simulink model "Ventilator_Controller"  (R2019b)
settings: Solver=ode23tb  StartTime=0  StopTime=1000  FixedStep=0.001  MaxStep=time_step_new  RelTol=0.01  EnableMultiTasking=on
values from neighbouring files (symbols this model uses):
  A = 20.9    [Gas_Exchange_IC.m]    (also in getPneumonia.m = (LF1-LF2)/(1-exp(Rresolve*(t2(end)-t2(1)))))
  a1 = 0.3836    [Dissociation_Spencer_IC.m]    (also in Gas_Exchange_IC.m; Respiratory_IC.m)
  a2 = 1.819    [Dissociation_Spencer_IC.m]    (also in Gas_Exchange_IC.m; Respiratory_IC.m)
  alpha1 = 0.02598    [Dissociation_Spencer_IC.m]    (also in Gas_Exchange_IC.m; Respiratory_IC.m)
  alpha2 = 0.05591    [Dissociation_Spencer_IC.m]    (also in Gas_Exchange_IC.m; Respiratory_IC.m)
  B = 92.8    [Gas_Exchange_IC.m]    (also in getPneumonia.m = LungFunction(end)-A)
  beta1 = 0.012275    [Dissociation_Spencer_IC.m]    (also in Gas_Exchange_IC.m; Respiratory_IC.m)
  beta2 = 0.03255    [Dissociation_Spencer_IC.m]    (also in Gas_Exchange_IC.m; Respiratory_IC.m)
  C = 10570    [Gas_Exchange_IC.m]
  C1 = 9    [Dissociation_Spencer_IC.m]    (also in Gas_Exchange_IC.m; Respiratory_IC.m)
  C2 = 87.00    (= 87)    [Dissociation_Spencer_IC.m]    (also in Gas_Exchange_IC.m; Respiratory_IC.m)
  Circadian_Period = 24    [Respiratory_IC.m]    (also in State_UA_Khoo_IC.m)
  CvCO2IC = 0.5116    [Body_Khoo_IC.m]    (also in Gas_Exchange_IC.m; Respiratory_IC.m = 0.5247)
  CvO2IC = 0.1672    [Body_Khoo_IC.m]    (also in Gas_Exchange_IC.m; Respiratory_IC.m = 0.1639)
  D = -5.251    [Gas_Exchange_IC.m]
  Dead1CO2IC = 0.1020    (= 0.102)    [Dead_Space_Khoo_IC.m]    (also in Gas_Exchange_IC.m; Respiratory_IC.m = 39.5616)
  Dead1O2IC = 149.8824    [Dead_Space_Khoo_IC.m]    (also in Gas_Exchange_IC.m; Respiratory_IC.m = 104.3637)
  Dead2CO2IC = 0.5274    [Dead_Space_Khoo_IC.m]    (also in Gas_Exchange_IC.m; Respiratory_IC.m = 39.6736)
  Dead2O2IC = 149.3923    [Dead_Space_Khoo_IC.m]    (also in Gas_Exchange_IC.m; Respiratory_IC.m = 104.2258)
  Dead3CO2IC = 2.2996    [Dead_Space_Khoo_IC.m]    (also in Gas_Exchange_IC.m; Respiratory_IC.m = 39.8127)
  Dead3O2IC = 147.3503    [Dead_Space_Khoo_IC.m]    (also in Gas_Exchange_IC.m; Respiratory_IC.m = 104.0505)
  Dead4CO2IC = 8.2293    [Dead_Space_Khoo_IC.m]    (also in Gas_Exchange_IC.m; Respiratory_IC.m = 40.0061)
  Dead4O2IC = 140.5179    [Dead_Space_Khoo_IC.m]    (also in Gas_Exchange_IC.m; Respiratory_IC.m = 103.8005)
  Dead5CO2IC = 22.0757    [Dead_Space_Khoo_IC.m]    (also in Gas_Exchange_IC.m; Respiratory_IC.m = 40.3359)
  Dead5O2IC = 124.5641    [Dead_Space_Khoo_IC.m]    (also in Gas_Exchange_IC.m; Respiratory_IC.m = 103.3579)
  DtotalIC = 0.3    [NeuroMuscular_IC.m]    (also in Respiratory_IC.m = 0.32)
  E_CW = 5    [Pleural_Schuessler_IC.m]    (also in Pmus_Flow_Younes_IC.m; Resp_Mech_IC.m; Respiratory_IC.m)
  E_L = 5    [Pleural_Schuessler_IC.m]    (also in Pmus_Flow_Younes_IC.m; Resp_Mech_IC.m; Respiratory_IC.m)
  fc = 0.4/60    (= 0.00666666666667)    [Respiratory_IC.m]    (also in State_UA_Khoo_IC.m)
  fcs_max = 47.78    [Cardiovascular_IC.m]    (also in Reflex_Ursino_IC.m)
  fcs_min = 2.52    [Cardiovascular_IC.m]    (also in Reflex_Ursino_IC.m)
  fcs_zero = 25    [Respiratory_IC.m]
  FlowIC = 0    [Pmus_Flow_Younes_IC.m]    (also in Resp_Mech_IC.m; Respiratory_IC.m)
  fp_inf = 6.3    [Respiratory_IC.m]
  fp_zero = 3.2    [Respiratory_IC.m]
  fs_inf = 2.10    (= 2.1)    [Respiratory_IC.m]
  fs_zero = 16.11    [Respiratory_IC.m]
  ftbs_min = 0.1    [Cardiovascular_IC.m]    (also in SA_Node_Ursino_IC.m)
  gc = 0.008/60    (= 0.000133333333333)    [Respiratory_IC.m]    (also in State_UA_Khoo_IC.m)
  h = 0.0183    [Brain_Khoo_IC.m]    (also in Gas_Exchange_IC.m; Respiratory_IC.m)
  HP_basal = 0.58    [Cardiovascular_IC.m]    (also in SA_Node_Ursino_IC.m)
  Ic = 45    [Gas_Exchange_IC.m]    (also in Respiratory_IC.m; Vent_Drive_Khoo_IC.m)
  IpCO2 = 38    [Gas_Exchange_IC.m]    (also in Respiratory_IC.m; Vent_Drive_Khoo_IC.m)
  IpO2 = 102.4    [Gas_Exchange_IC.m]    (also in Respiratory_IC.m; Vent_Drive_Khoo_IC.m)
  K1 = 13    [Dissociation_Spencer_IC.m]    (also in Gas_Exchange_IC.m; Respiratory_IC.m)
  K2 = 194.4    [Dissociation_Spencer_IC.m]    (also in Gas_Exchange_IC.m; Respiratory_IC.m)
  k_cs = 11.758    [Cardiovascular_IC.m]    (also in Reflex_Ursino_IC.m)
  k_p = 7.06    [Respiratory_IC.m]
  k_s = 0.07    [Respiratory_IC.m]
  lambda = 863    [Gas_Exchange_IC.m]    (also in Lungs_Khoo_IC.m; Respiratory_IC.m)
  Mech_Vent_pressure = 17    [Mech_vent_test.m]
  MRbCO2 = 0.0517    [Brain_Khoo_IC.m]    (also in Gas_Exchange_IC.m; Respiratory_IC.m)
  MRCO2 = 0.0033    [Body_Khoo_IC.m]    (also in Gas_Exchange_IC.m; Respiratory_IC.m)
  MRO2 = 0.0038    [Body_Khoo_IC.m]    (also in Gas_Exchange_IC.m; Respiratory_IC.m)
  NM_block_gain = 1    [Mech_vent_test.m]
  PACO2_delayIC = 39.6041    [Cardio_Mix_Lange_IC.m]    (also in Gas_Exchange_IC.m; Respiratory_IC.m = 40.4448)
  PaCO2firstIC = 0.2150    (= 0.215)    [Cardio_Mix_Lange_IC.m]    (also in Gas_Exchange_IC.m; Respiratory_IC.m = -0.2465)
  PACO2IC = 37.1484    [Gas_Exchange_IC.m]    (also in Lungs_Khoo_IC.m; Respiratory_IC.m = 40.9432)
  PaCO2secondIC = 38.4577    [Cardio_Mix_Lange_IC.m]    (also in Gas_Exchange_IC.m; Respiratory_IC.m = 40.3928)
  PAO2_delayIC = 103.8436    [Cardio_Mix_Lange_IC.m]    (also in Gas_Exchange_IC.m; Respiratory_IC.m = 103.1223)
  PaO2firstIC = -0.2838    [Cardio_Mix_Lange_IC.m]    (also in Gas_Exchange_IC.m; Respiratory_IC.m = 0.3557)
  PAO2IC = 107.1983    [Gas_Exchange_IC.m]    (also in Lungs_Khoo_IC.m; Respiratory_IC.m = 102.5153)
  PaO2secondIC = 105.4828    [Cardio_Mix_Lange_IC.m]    (also in Gas_Exchange_IC.m; Respiratory_IC.m = 103.1435)
  PbCO2IC = 48.2858    [Brain_Khoo_IC.m]    (also in Gas_Exchange_IC.m; Respiratory_IC.m = 48.5383)
  PICO2 = 0    [Dead_Space_Khoo_IC.m]    (also in Gas_Exchange_IC.m; Respiratory_IC.m)
  PICO2_change = 0    [Respiratory_IC.m]
  PIO2 = 150    [Dead_Space_Khoo_IC.m]    (also in Gas_Exchange_IC.m; Respiratory_IC.m)
  PIO2_change = -90    [Mech_vent_test.m]    (also in Respiratory_IC.m = 0)
  Pn = 90    [Cardiovascular_IC.m]    (also in Reflex_Ursino_IC.m)
  Pt_frcIC1 = 0    [Pmus_Flow_Younes_IC.m]    (also in Resp_Mech_IC.m; Respiratory_IC.m)
  Pt_frcIC2 = 0    [Pmus_Flow_Younes_IC.m]    (also in Resp_Mech_IC.m; Respiratory_IC.m)
  QdBo = 0.8333    [Brain_Khoo_IC.m]    (also in Gas_Exchange_IC.m; Respiratory_IC.m)
  R_AW = 1.27    [Pleural_Schuessler_IC.m]    (also in Pmus_Flow_Younes_IC.m; Resp_Mech_IC.m; Respiratory_IC.m)
  R_CW = 1.03    [Pleural_Schuessler_IC.m]    (also in Pmus_Flow_Younes_IC.m; Resp_Mech_IC.m; Respiratory_IC.m)
  R_L = 1.69    [Pleural_Schuessler_IC.m]    (also in Pmus_Flow_Younes_IC.m; Resp_Mech_IC.m; Respiratory_IC.m)
  RC = 0.06    [Pleural_Schuessler_IC.m]    (also in Pmus_Flow_Younes_IC.m; Resp_Mech_IC.m; Respiratory_IC.m)
  rc = 0.2/60    (= 0.00333333333333)    [Respiratory_IC.m]    (also in State_UA_Khoo_IC.m)
  SbCO2 = 0.3600    (= 0.36)    [Brain_Khoo_IC.m]    (also in Gas_Exchange_IC.m; Respiratory_IC.m)
  SCO2 = 0.0043    [Brain_Khoo_IC.m]    (also in Gas_Exchange_IC.m; Respiratory_IC.m)
  SWAo = 0.007    [Respiratory_IC.m]    (also in State_UA_Khoo_IC.m)
  T1 = 1    [Cardio_Mix_Lange_IC.m]    (also in Gas_Exchange_IC.m; Respiratory_IC.m)
  T2 = 2    [Cardio_Mix_Lange_IC.m]    (also in Gas_Exchange_IC.m; Respiratory_IC.m)
  t_CO2_duration = 0    [Respiratory_IC.m]
  t_CO2_start = 0    [Respiratory_IC.m]
  t_end_new = 4*24*60*60    (= 345600)    [Mech_vent_test.m]
  t_end_UA = 0    [Respiratory_IC.m]    (also in State_UA_Khoo_IC.m)
  t_Mech_Vent_duration = 0    [Mech_vent_test.m]
  t_Mech_Vent_start = 0    [Mech_vent_test.m]
  t_Mueller_duration = 0    [NeuroMuscular_IC.m]
  t_Mueller_insp = 0    [NeuroMuscular_IC.m]
  t_Mueller_start = 0    [NeuroMuscular_IC.m]
  t_NM_block_duration = 0    [Mech_vent_test.m]
  t_NM_block_start = 0    [Mech_vent_test.m]
  t_O2_duration = 0    [Mech_vent_test.m]    (also in Respiratory_IC.m)
  t_O2_start = 0    [Mech_vent_test.m]    (also in Respiratory_IC.m)
  t_start_new = 0    [Mech_vent_test.m]
  t_start_UA = 0    [Respiratory_IC.m]    (also in State_UA_Khoo_IC.m)
  t_valsalva_duration = 0    [NeuroMuscular_IC.m]
  t_valsalva_insp = 0    [NeuroMuscular_IC.m]
  t_valsalva_start = 0    [NeuroMuscular_IC.m]
  time_step = time_step    [acquire_data.m]    (also in acquire_data_save.m)
  VC = 5    [Pmus_Flow_Younes_IC.m]    (also in Resp_Mech_IC.m; Respiratory_IC.m)
  Vdead1 = 0.03    [Dead_Space_Khoo_IC.m]    (also in Gas_Exchange_IC.m; Respiratory_IC.m)
  Vdead2 = 0.03    [Dead_Space_Khoo_IC.m]    (also in Gas_Exchange_IC.m; Respiratory_IC.m)
  Vdead3 = 0.03    [Dead_Space_Khoo_IC.m]    (also in Gas_Exchange_IC.m; Respiratory_IC.m)
  Vdead4 = 0.03    [Dead_Space_Khoo_IC.m]    (also in Gas_Exchange_IC.m; Respiratory_IC.m)
  Vdead5 = 0.03    [Dead_Space_Khoo_IC.m]    (also in Gas_Exchange_IC.m; Respiratory_IC.m)
  Ventilator_rate = 12    [Mech_vent_test.m]
  VTCO2 = 15    [Body_Khoo_IC.m]    (also in Gas_Exchange_IC.m; Respiratory_IC.m)
  VtIC = 0    [Pmus_Flow_Younes_IC.m]    (also in Resp_Mech_IC.m; Respiratory_IC.m)
  VTO2 = 6    [Body_Khoo_IC.m]    (also in Gas_Exchange_IC.m; Respiratory_IC.m)
  Z = 0.0227    [Dissociation_Spencer_IC.m]    (also in Gas_Exchange_IC.m; Respiratory_IC.m)
undefined symbols (not defined in the file or in its folder): A_0_ua, alpha_E_FFA_Heart, alpha_E_FFA_muscle, alpha_E_GLC_Heart, alpha_E_GLC_muscle, alpha_E_GLY_muscle, alpha_E_PYR_muscle, alpha_E_TGL_adipose, alpha_E_TGL_GI, alpha_E_TGL_Heart, alpha_E_TGL_muscle, Arousal_UAIC, C_ua_awake, Cbp, Cbv, Ce_0, Cep, Cev, Chp, Chv, Cla, Clamp_class, Cmp, Cmv, Cpa, CPAP_pressure, Cpp, Cpv, Cra, Csa, Csp, Csv, CvbO2_n, CvhO2_n, CvmO2_n, DAY, delay, DietBlock, Dx, Fb, fchemo_max, fchemo_min, fchemoIC, flsIC, Ftas_I0, ftas_min, ftas_r0, FVC_activation, gain_E, Gamma, Gas_sleep, Gas_sleepM, Gb, Gblock, GbO2, Gbs_sleep, gcc_sa, gcc_sb, gcc_sp, Gclamp ... (+147)
libraries: simulink x4, simulink_extras x2
(part 1 of 8)
settings Model: SimulationMode=accelerator  ExtModeTrigMode=oneshot  ExtModeArmWhenConnect=off  Creator=cPhonix  LastModifiedBy=z9070419
settings SolverCC: MaxConsecutiveZCs=10000  AutoInsertRateTranBlk=on
settings DataIOCC: FinalStateName=yFinal  InitialState=xFinal  SaveFormat=Array  SaveOutput=off  SaveTime=off  ReturnWorkspaceOutputs=off  TimeSaveName=T_SIMULATION  SignalLoggingName=sigsOut
settings OptimizationCC: BlockReduction=off  BooleanDataType=off  ExpressionDepthLimit=2147483647  InitFltsAndDblsToZero=on  LifeSpan=inf
settings DebuggingCC: AlgebraicLoopMsg=error  ArtificialAlgebraicLoopMsg=error  SaveWithParameterizedLinksMsg=none  UnderspecifiedInitializationDetection=Classic  MergeDetectMultiDrivingBlocksExec=none  SignalResolutionControl=TryResolveAllWithWarning  InheritedTsInSrcMsg=none  MultiTaskDSMMsg=warning  MultiTaskCondExecSysMsg=none  MultiTaskRateTransMsg=warning  TasksWithSamePriorityMsg=none  SigSpecEnsureSampleTimeMsg=none  IntegerOverflowMsg=none  Int32ToFloatConvMsg=none  ParameterDowncastMsg=warning  ParameterOverflowMsg=none  FcnCallInpInsideContextMsg=warning  ModelReferenceDataLoggingMessage=none  StateNameClashWarn=warning  SFUnexpectedBacktrackingDiag=warning  SFNoUnconditionalDefaultTransitionDiag=warning  SFExecutionAtInitializationDiag=none  IntegerSaturationMsg=none  ArithmeticOperatorsInVariantConditions=warning
settings HardwareCC: ProdBitPerPointer=32  ProdBitPerSizeT=32  ProdBitPerPtrDiffT=32  ProdLargestAtomicFloat=None  ProdIntDivRoundTo=Undefined  ProdEndianess=Unspecified  ProdWordSize=32  ProdHWDeviceType=32-bit Generic  TargetBitPerPointer=64  TargetBitPerSizeT=64  TargetBitPerPtrDiffT=64  TargetLongLongMode=on  TargetIntDivRoundTo=Zero  TargetEndianess=LittleEndian  TargetWordSize=64  TargetHWDeviceType=MATLAB Host  ProdEqTarget=off
settings ModelReferenceCC: PropagateSignalLabelsOutOfModel=off
settings SFSimCC: SimParseCustomCode=off
settings CodeAppCC: StateflowObjectComments=on
settings GRTTargetCC: TargetLangStandard=C89/C90 (ANSI)  CombineOutputUpdateFcns=off  GRTInterface=on
settings ConfigComp: CovMetricSettings=dw  CovHtmlReporting=on  CovSaveCumulativeToWorkspaceVar=on  CovSaveSingleToWorkspaceVar=on

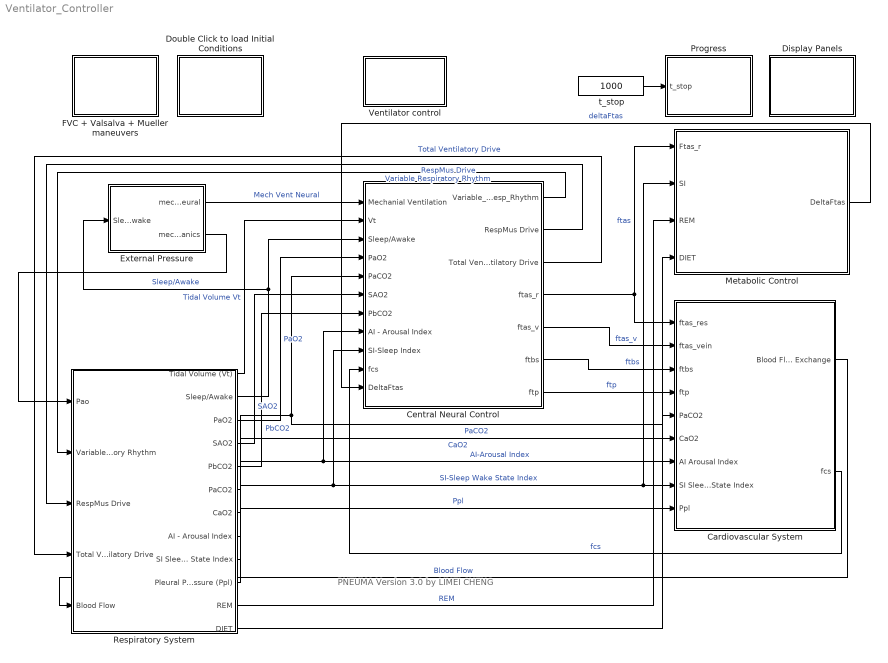
== system Ventilator_Controller ==
  note: PNEUMA Version 3.0 by LIMEI CHENG
  Cardiovascular System : Subsystem
      mask Display: image(imread('CV_pic.bmp'))
  Central Neural Control : Subsystem
      mask Display: image(imread('CNS.bmp'))
  Display Panels : Subsystem
      mask Display: disp('Display \nPanel','b')
  Double Click to load Initial Conditions : Subsystem
      settings: OpenFcn=pneuma_variables
      mask Display: image(imread('IC_pic.bmp'))
  External Pressure : Subsystem
      mask Display: image(imread('CPAP2.bmp'))
  FVC + Valsalva + Mueller maneuvers : Subsystem
      mask Display: disp('Maneuvers')
  Metabolic Control : Subsystem
      mask Display: image(imread('Metabolic2.bmp'))
  Progress : Subsystem
      mask Display: disp('Progress')
  Respiratory System : Subsystem
      mask Display: image(imread('Respiratory_System.bmp'))
  Ventilator control : Subsystem
  t_stop : Constant  Value=1000
  wires:
  Central Neural Control/3(Total Ventilatory Drive) -> Respiratory System/4(Total Ventilatory Drive)  "Total Ventilatory Drive"
  Central Neural Control/2(RespMus Drive) -> Respiratory System/3(RespMus Drive)  "RespMus Drive"
  External Pressure/1(mech vent neural) -> Central Neural Control/1(Mechanial Ventilation)  "Mech Vent Neural"
  Cardiovascular System/1(Blood Flow to Lung for Gas Exchange) -> Respiratory System/5(Blood Flow)  "Blood Flow"
  Cardiovascular System/2(fcs) -> Central Neural Control/10(fcs)  "fcs"
  t_stop/1 -> Progress/1(t_stop)
  Central Neural Control/1(Variable_Resp_Rhythm) -> Respiratory System/2(Variable Respiratory Rhythm)  "Variable Respiratory Rhythm"
  Respiratory System/1(Tidal Volume (Vt)) -> Central Neural Control/2(Vt)  "Tidal Volume Vt"
  Respiratory System/2(Sleep/Awake) -> Central Neural Control/3(Sleep/Awake), External Pressure/1(SleepAwake)  "Sleep/Awake"
  Respiratory System/3(PaO2) -> Central Neural Control/4(PaO2)  "PaO2"
  Respiratory System/6(PaCO2) -> Central Neural Control/5(PaCO2), Cardiovascular System/5(PaCO2)  "PaCO2"
  Respiratory System/4(SAO2) -> Central Neural Control/6(SAO2)  "SAO2"
  Respiratory System/5(PbCO2) -> Central Neural Control/7(PbCO2)  "PbCO2"
  Respiratory System/8(AI - Arousal Index) -> Central Neural Control/8(AI - Arousal Index), Cardiovascular System/7(AI Arousal Index)  "AI-Arousal Index"
  Respiratory System/9(SI Sleep Wake State Index) -> Metabolic Control/2(SI), Cardiovascular System/8(SI Sleep-Wake State Index), Central Neural Control/9(SI-Sleep Index)  "SI-Sleep Wake State Index"
  Respiratory System/10(Pleural Pressure (Ppl)) -> Cardiovascular System/9(Ppl)  "Ppl"
  External Pressure/2(mech vent mechanics) -> Respiratory System/1(Pao)
  Respiratory System/7(CaO2) -> Cardiovascular System/6(CaO2)  "CaO2"
  Central Neural Control/4(ftas_r) -> Metabolic Control/1(Ftas_r), Cardiovascular System/1(ftas_res)  "ftas"
  Central Neural Control/5(ftas_v) -> Cardiovascular System/2(ftas_vein)  "ftas_v"
  Central Neural Control/6(ftbs) -> Cardiovascular System/3(ftbs)  "ftbs"
  Central Neural Control/7(ftp) -> Cardiovascular System/4(ftp)  "ftp"
  Respiratory System/11(REM) -> Metabolic Control/3(REM)  "REM"
  Metabolic Control/1(DeltaFtas) -> Central Neural Control/11(DeltaFtas)  "deltaFtas"
  Respiratory System/12(DIET) -> Metabolic Control/4(DIET)

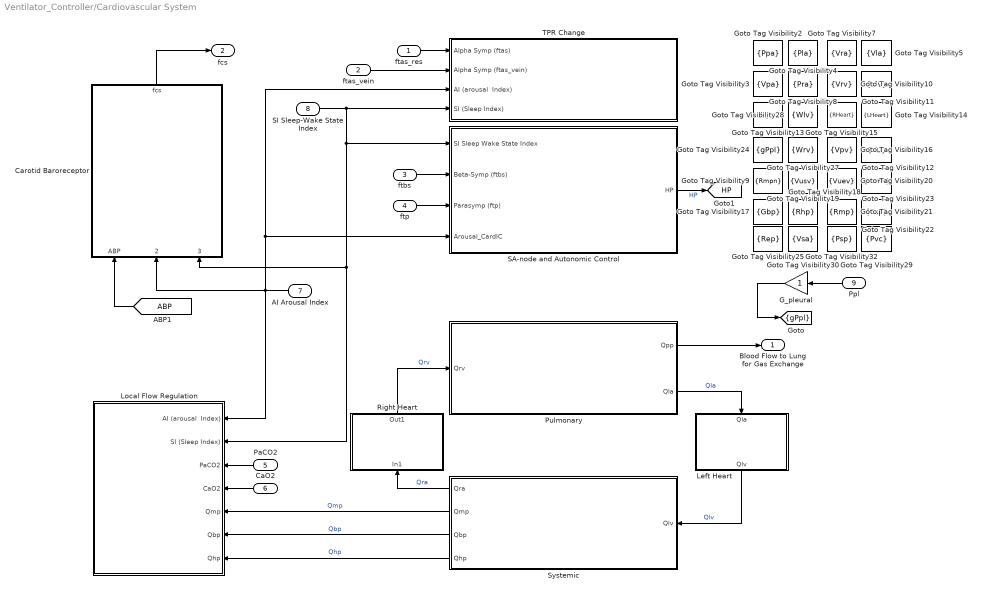
== system Ventilator_Controller/Cardiovascular System ==
  ftas_res : Inport
  ftas_vein : Inport  Port=2
  ftbs : Inport  Port=3
  ftp : Inport  Port=4
  PaCO2 : Inport  Port=5
  CaO2 : Inport  Port=6
  AI Arousal Index : Inport  Port=7  OutDataTypeStr=double
  SI Sleep-Wake State Index : Inport  Port=8
  Ppl : Inport  Port=9
  Carotid Baroreceptor : Subsystem
      mask Display: disp('Carotid\n Baroreceptor')
  G_pleural : Gain  SaturateOnIntegerOverflow=on  OutDataTypeStr=Inherit: Same as input  ParamDataTypeStr=Inherit: Same as input
  Goto Tag Visibility10 : GotoTagVisibility  GotoTag=Vrv
  Goto Tag Visibility11 : GotoTagVisibility  GotoTag=Vlv
  Goto Tag Visibility12 : GotoTagVisibility  GotoTag=Vu
  Goto Tag Visibility13 : GotoTagVisibility  GotoTag=Vpp
  Goto Tag Visibility14 : GotoTagVisibility  GotoTag=LHeart
  Goto Tag Visibility15 : GotoTagVisibility  GotoTag=RHeart
  Goto Tag Visibility16 : GotoTagVisibility  GotoTag=Vpv
  Goto Tag Visibility17 : GotoTagVisibility  GotoTag=Gbp
  Goto Tag Visibility18 : GotoTagVisibility  GotoTag=Rhp
  Goto Tag Visibility19 : GotoTagVisibility  GotoTag=Vusv
  Goto Tag Visibility2 : GotoTagVisibility  GotoTag=Ppa
  Goto Tag Visibility20 : GotoTagVisibility  GotoTag=Vuev
  Goto Tag Visibility21 : GotoTagVisibility  GotoTag=Rmp
  Goto Tag Visibility22 : GotoTagVisibility  GotoTag=Rsp
  Goto Tag Visibility23 : GotoTagVisibility  GotoTag=Vumv
  Goto Tag Visibility24 : GotoTagVisibility  GotoTag=gPpl
  Goto Tag Visibility25 : GotoTagVisibility  GotoTag=Rep
  Goto Tag Visibility27 : GotoTagVisibility  GotoTag=Wrv
  Goto Tag Visibility28 : GotoTagVisibility  GotoTag=Wlv
  Goto Tag Visibility29 : GotoTagVisibility  GotoTag=Pvc
  Goto Tag Visibility3 : GotoTagVisibility  GotoTag=Vpa
  Goto Tag Visibility30 : GotoTagVisibility  GotoTag=Vsa
  Goto Tag Visibility32 : GotoTagVisibility  GotoTag=Psp
  Goto Tag Visibility4 : GotoTagVisibility  GotoTag=Pla
  Goto Tag Visibility5 : GotoTagVisibility  GotoTag=Vla
  Goto Tag Visibility7 : GotoTagVisibility  GotoTag=Vra
  Goto Tag Visibility8 : GotoTagVisibility  GotoTag=Pra
  Goto Tag Visibility9 : GotoTagVisibility  GotoTag=Rmpn
  Left Heart : Subsystem
      mask Display: disp('LEFT HEART')
  Local Flow Regulation : Subsystem
      mask Display: disp('Local Flow Regulation')
  Pulmonary : Subsystem
      mask Display: disp('PULMONARY CIRCULATORY SYSTEM')
  Right Heart : Subsystem
      mask Display: disp('RIGHT HEART')
  SA-node and Autonomic Control : Subsystem
  Systemic : Subsystem
      mask Display: disp('SYSTEMIC CIRULATORY SYSTEM')
  TPR Change : Subsystem
  Blood Flow to Lung for Gas Exchange : Outport
  fcs : Outport  Port=2
  tag scope: HP=global, gPpl=scoped
  wires:
  ftp/1 -> SA-node and Autonomic Control/3(Parasymp (ftp))
  ftbs/1 -> SA-node and Autonomic Control/2(Beta-Symp (ftbs))
  ftas_res/1 -> TPR Change/1(Alpha Symp (ftas))
  Carotid Baroreceptor/1(fcs) -> fcs/1
  SI Sleep-Wake State Index/1 -> SA-node and Autonomic Control/1(SI Sleep Wake State Index), Carotid Baroreceptor/3(SI Sleep Wake State Index), Local Flow Regulation/2("SI (Sleep Index) "), TPR Change/4("SI (Sleep Index) ")
  Ppl/1 -> G_pleural/1
  G_pleural/1 -> [gPpl]
  SA-node and Autonomic Control/1(HP) -> [HP]  "HP"
  [ABP] -> Carotid Baroreceptor/1(ABP)
  Systemic/1(Qra) -> Right Heart/1(In1)  "Qra"
  Left Heart/1(Qlv) -> Systemic/1(Qlv)  "Qlv"
  Right Heart/1(Out1) -> Pulmonary/1(Qrv)  "Qrv"
  Pulmonary/2(Qla) -> Left Heart/1(Qla)  "Qla"
  ftas_vein/1 -> TPR Change/2(Alpha Symp (ftas_vein))
  PaCO2/1 -> Local Flow Regulation/3(PaCO2)
  CaO2/1 -> Local Flow Regulation/4(CaO2)
  Systemic/2(Qmp) -> Local Flow Regulation/5(Qmp)  "Qmp"
  Systemic/3(Qbp) -> Local Flow Regulation/6(Qbp)  "Qbp"
  Systemic/4(Qhp) -> Local Flow Regulation/7(Qhp)  "Qhp"
  Pulmonary/1(Qpp) -> Blood Flow to Lung for Gas Exchange/1
  AI Arousal Index/1 -> Carotid Baroreceptor/2("AI - Arousal Index "), SA-node and Autonomic Control/4(Arousal_CardIC), TPR Change/3(AI (arousal  Index)), Local Flow Regulation/1(AI (arousal  Index))

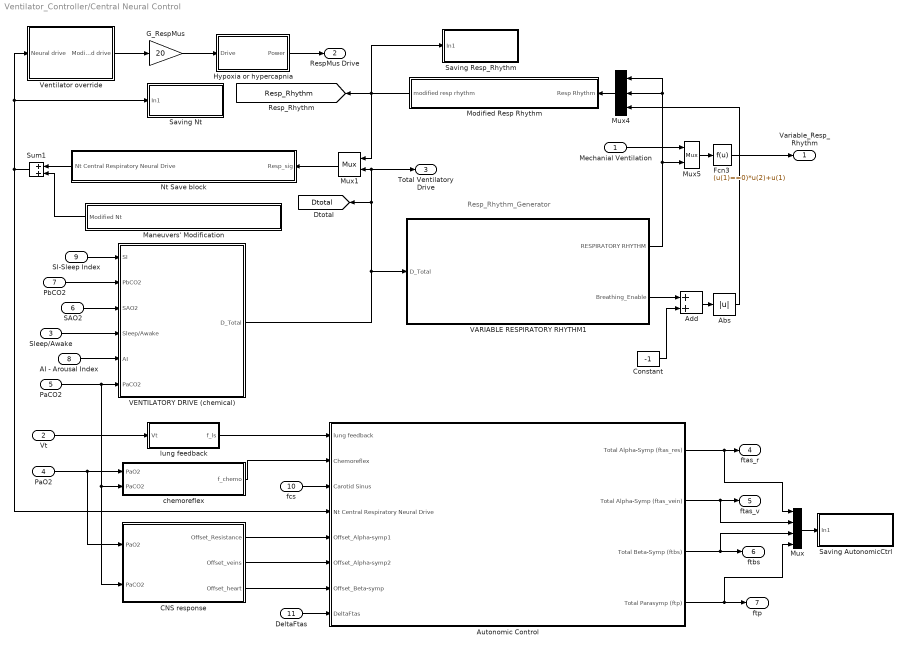
== system Ventilator_Controller/Central Neural Control ==
  note: Resp_Rhythm_Generator
  Mechanial Ventilation : Inport
  Vt : Inport  Port=2
  Sleep/Awake : Inport  Port=3
  PaO2 : Inport  Port=4
  PaCO2 : Inport  Port=5
  SAO2 : Inport  Port=6
  PbCO2 : Inport  Port=7
  AI - Arousal Index : Inport  Port=8
  SI-Sleep Index : Inport  Port=9
  fcs : Inport  Port=10
  DeltaFtas : Inport  Port=11
  Abs : Abs
  Add : Sum
  Autonomic Control : Subsystem
  CNS response : Subsystem
  Constant : Constant  Value=-1
  Fcn3 : Fcn  Expr=(u(1)==0)*u(2)+u(1)
  G_RespMus : Gain  Gain=20  SaturateOnIntegerOverflow=on  OutDataTypeStr=Inherit: Same as input  ParamDataTypeStr=Inherit: Same as input
  Hypoxia or hypercapnia : Subsystem
  Maneuvers' Modification : Subsystem
  Modified Resp Rhythm : Subsystem
  Mux : Mux
  Mux1 : Mux  Inputs=2
  Mux4 : Mux  Inputs=3
  Mux5 : Mux  Inputs=2
  Nt Save block : Subsystem
  Saving AutonomicCtrl : Subsystem
  Saving Nt : Subsystem
  Saving Resp_Rhythm : Subsystem
  Sum1 : Sum  SaturateOnIntegerOverflow=on  InputSameDT=on  OutDataTypeStr=Inherit: Same as first input
  VARIABLE RESPIRATORY RHYTHM1 : Subsystem
  VENTILATORY DRIVE (chemical) : Subsystem
  Ventilator override : Subsystem
  chemoreflex : Subsystem
  lung feedback : Subsystem
  Variable_Resp_Rhythm : Outport
  RespMus Drive : Outport  Port=2
  Total Ventilatory Drive : Outport  Port=3
  ftas_r : Outport  Port=4
  ftas_v : Outport  Port=5
  ftbs : Outport  Port=6
  ftp : Outport  Port=7
  tag scope: Dtotal=global, Resp_Rhythm=global
  wires:
  Mechanial Ventilation/1 -> Mux5/1
  Nt Save block/1(Nt Central Respiratory Neural Drive) -> Sum1/1
  Mux1/1 -> Nt Save block/1(Resp_sig)
  Modified Resp Rhythm/1("modified resp rhythm ") -> [Resp_Rhythm], Saving Resp_Rhythm/1(In1), Mux1/1
  lung feedback/1(f_ls) -> Autonomic Control/1(lung feedback)
  chemoreflex/1(f_chemo) -> Autonomic Control/2(Chemoreflex)
  Autonomic Control/1(Total Alpha-Symp (ftas_res)) -> ftas_r/1, Mux/1
  Autonomic Control/3(Total Beta-Symp (ftbs)) -> ftbs/1, Mux/3
  Autonomic Control/4(Total Parasymp (ftp)) -> Mux/4, ftp/1
  PaCO2/1 -> VENTILATORY DRIVE (chemical)/6(PaCO2), chemoreflex/2(PaCO2), CNS response/2(PaCO2)
  Vt/1 -> lung feedback/1(Vt)
  PaO2/1 -> chemoreflex/1(PaO2), CNS response/1(PaO2)
  fcs/1 -> Autonomic Control/3(Carotid Sinus)
  SAO2/1 -> VENTILATORY DRIVE (chemical)/3(SAO2)
  Sleep/Awake/1 -> VENTILATORY DRIVE (chemical)/4(Sleep/Awake)
  PbCO2/1 -> VENTILATORY DRIVE (chemical)/2(PbCO2)
  Mux4/1 -> Modified Resp Rhythm/1(Resp Rhythm)
  Add/1 -> Abs/1
  VARIABLE RESPIRATORY RHYTHM1/2(Breathing_Enable) -> Add/1
  Constant/1 -> Add/2
  Abs/1 -> Mux4/3
  Sum1/1 -> Autonomic Control/4(Nt Central Respiratory Neural Drive), Saving Nt/1(In1), Ventilator override/1(Neural drive)
  Maneuvers' Modification/1(Modified Nt) -> Sum1/2
  Mux5/1 -> Fcn3/1
  Fcn3/1 -> Variable_Resp_Rhythm/1
  AI - Arousal Index/1 -> VENTILATORY DRIVE (chemical)/5(AI)
  Autonomic Control/2(Total Alpha-Symp (ftas_vein)) -> ftas_v/1, Mux/2
  SI-Sleep Index/1 -> VENTILATORY DRIVE (chemical)/1(SI)
  CNS response/1(Offset_Resistance) -> Autonomic Control/5(Offset_Alpha-symp1)
  CNS response/2(Offset_veins) -> Autonomic Control/6(Offset_Alpha-symp2)
  CNS response/3(Offset_heart) -> Autonomic Control/7(Offset_Beta-symp)
  Mux/1 -> Saving AutonomicCtrl/1(In1)
  VENTILATORY DRIVE (chemical)/1(D_Total) -> Mux1/2, Total Ventilatory Drive/1, [Dtotal], VARIABLE RESPIRATORY RHYTHM1/1(D_Total)
  VARIABLE RESPIRATORY RHYTHM1/1(RESPIRATORY RHYTHM) -> Mux5/2, Mux4/2, Mux4/1
  DeltaFtas/1 -> Autonomic Control/8(DeltaFtas)
  Ventilator override/1("Modified drive ") -> G_RespMus/1
  G_RespMus/1 -> Hypoxia or hypercapnia/1(Drive)
  Hypoxia or hypercapnia/1(Power) -> RespMus Drive/1

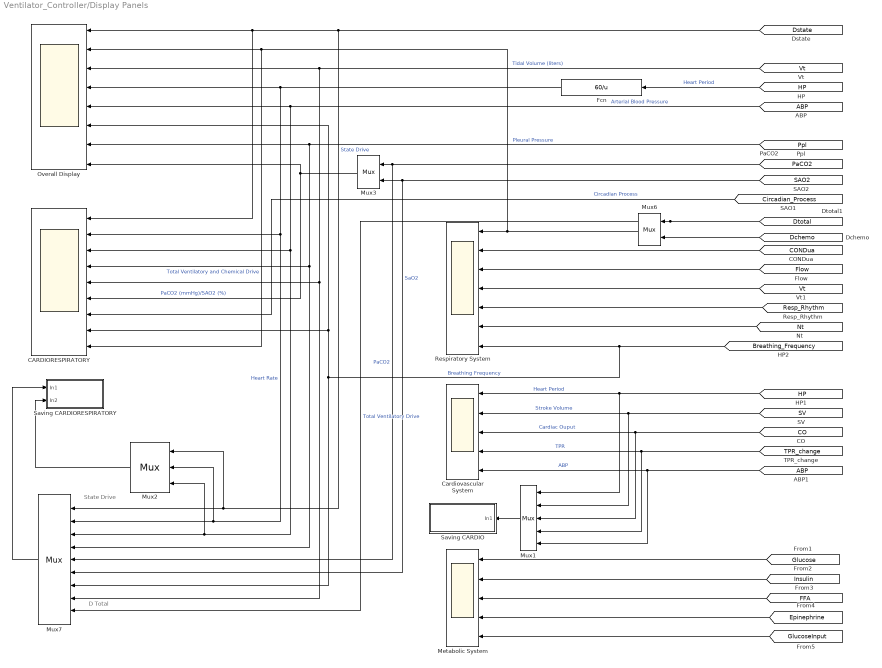
== system Ventilator_Controller/Display Panels ==
  note: D Total
  note: State Drive
  CARDIORESPIRATORY : Scope  NumInputPorts=9
  Cardiovascular System : Scope  NumInputPorts=5
  Fcn : Fcn  Expr=60/u
  Metabolic System : Scope  NumInputPorts=5
  Mux1 : Mux  Inputs=5
  Mux2 : Mux  Inputs=3
  Mux3 : Mux  Inputs=2
  Mux6 : Mux  Inputs=2
  Mux7 : Mux  Inputs=9
  Overall Display : Scope  NumInputPorts=8
  Respiratory System : Scope  NumInputPorts=7
  Saving CARDIORESPIRATORY : Subsystem
  Saving CARDIO : Subsystem
  wires:
  Mux3/1 -> Overall Display/8, CARDIORESPIRATORY/6  "PaCO2 (mmHg)/SAO2 (%)"
  [Vt] -> Overall Display/3, CARDIORESPIRATORY/5, Mux7/8  "Tidal Volume (liters)"
  [ABP] -> Overall Display/5, CARDIORESPIRATORY/3, Mux7/3, Mux2/3  "Arterial Blood Pressure"
  [Ppl] -> Overall Display/7, CARDIORESPIRATORY/4, Mux7/4  "Pleural Pressure"
  [SAO2] -> Mux3/2, Mux7/6  "SaO2"
  [PaCO2] -> Mux3/1, Mux7/5  "PaCO2"
  [HP] -> Fcn/1  "Heart Period"
  Fcn/1 -> Overall Display/4, CARDIORESPIRATORY/2, Mux7/2, Mux2/2  "Heart Rate"
  [Dstate] -> Overall Display/1, CARDIORESPIRATORY/1, Mux7/1, Mux2/1  "State Drive"
  Mux6/1 -> Respiratory System/1, Overall Display/2, CARDIORESPIRATORY/9  "Total Ventilatory and Chemical Drive"
  [Resp_Rhythm] -> Respiratory System/5
  [Breathing_Frequency] -> Respiratory System/7, Overall Display/6, CARDIORESPIRATORY/8, Mux7/7  "Breathing Frequency"
  Mux7/1 -> Saving CARDIORESPIRATORY/1(In1)
  [Dtotal] -> Mux6/1, Mux7/9  "Total Ventilatory Drive"
  [Dchemo] -> Mux6/2
  [CONDua] -> Respiratory System/2
  [Flow] -> Respiratory System/3
  [Vt] -> Respiratory System/4
  [Nt] -> Respiratory System/6
  [HP] -> Cardiovascular System/1, Mux1/1  "Heart Period"
  [SV] -> Cardiovascular System/2, Mux1/2  "Stroke Volume"
  [CO] -> Cardiovascular System/3, Mux1/3  "Cardiac Ouput"
  [TPR_change] -> Cardiovascular System/4, Mux1/4  "TPR"
  [ABP] -> Cardiovascular System/5, Mux1/5  "ABP"
  [Circadian_Process] -> CARDIORESPIRATORY/7  "Circadian Process"
  Mux1/1 -> Saving CARDIO/1(In1)
  [Glucose] -> Metabolic System/1
  [Insulin] -> Metabolic System/2
  [FFA] -> Metabolic System/3
  [Epinephrine] -> Metabolic System/4
  [GlucoseInput] -> Metabolic System/5
  Mux2/1 -> Saving CARDIORESPIRATORY/2(In2)

== system Ventilator_Controller/Double Click to load Initial Conditions ==
  Mux : Mux  Inputs=32
      settings: DisplayOption=signals
  To File : ToFile  Filename=RespICSampled100.mat  MatrixName=RespIC_Sampled100  SampleTime=100
  wires:
  Mux/1 -> To File/1
  [Nt] -> Mux/1
  [Flow] -> Mux/2
  [Vt] -> Mux/3
  [Ppl] -> Mux/4
  [SAO2] -> Mux/5
  [PaCO2] -> Mux/6
  [CONDua] -> Mux/7
  [Dstate] -> Mux/8
  [Dchemo] -> Mux/9
  [Arousal_UAIC] -> Mux/10
  [Dtotal] -> Mux/11
  [Dead1CO2IC] -> Mux/12
  [Dead2CO2IC] -> Mux/13
  [Dead3CO2IC] -> Mux/14
  [Dead4CO2IC] -> Mux/15
  [Dead5CO2IC] -> Mux/16
  [Dead1O2IC] -> Mux/17
  [Dead2O2IC] -> Mux/18
  [Dead3O2IC] -> Mux/19
  [Dead4O2IC] -> Mux/20
  [Dead5O2IC] -> Mux/21
  [PACO2IC] -> Mux/22
  [PAO2IC] -> Mux/23
  [PaCO2firstIC] -> Mux/24
  [PaCO2secondIC] -> Mux/25
  [PaO2firstIC] -> Mux/26
  [PaO2secondIC] -> Mux/27
  [CvCO2IC] -> Mux/28
  [CvO2IC] -> Mux/29
  [PbCO2IC] -> Mux/30
  [PACO2_delayIC] -> Mux/31
  [PAO2_delayIC] -> Mux/32

== system Ventilator_Controller/External Pressure ==
  SleepAwake : Inport
  Annoxia or hypercapnia : Subsystem
  CPAP Control : Subsystem  mask{begin_time=t_CPAP_start, end_time=t_CPAP_start+t_CPAP_duration, init_value=0, final_value=1}
      mask prompts: begin_time "pulse begin"; end_time "pulse end"; init_value "initial value"; final_value "final value"
      mask Display: disp('pulse')
  CPAP Pressure : Subsystem  mask{begin_time=t_CPAP_start, end_time=t_CPAP_start+t_CPAP_duration, init_value=0, final_value=CPAP_pressure}
      mask prompts: begin_time "pulse begin"; end_time "pulse end"; init_value "initial value"; final_value "final value"
      mask Display: disp('pulse')
  CPAP_activation : Gain  Gain=0  SaturateOnIntegerOverflow=on  OutDataTypeStr=Inherit: Same as input  ParamDataTypeStr=Inherit: Same as input
  CPAP_pressure : Gain  Gain=CPAP_pressure  SaturateOnIntegerOverflow=on  OutDataTypeStr=Inherit: Same as input  ParamDataTypeStr=Inherit: Same as input
  Divide : Product  Inputs=**
  Fcn : Fcn  Expr=1-u
  Integrator : Integrator  ExternalReset=falling
  Manual Switch : ManualSwitch
  Math Function : Math  Operator=sqrt  SaturateOnIntegerOverflow=on
  Product : Product  RndMeth=Zero
  Product5 : Product  SaturateOnIntegerOverflow=on  InputSameDT=on  OutDataTypeStr=Inherit: Same as first input
  Sum5 : Sum  SaturateOnIntegerOverflow=on  InputSameDT=on  OutDataTypeStr=Inherit: Same as first input
  Transfer Fcn : TransferFcn  Numerator=[7]  Denominator=[1 2.2]
  mech vent neural : Outport
  mech vent mechanics : Outport  Port=2
  tag scope: MuscleContractility=global
  wires:
  Sum5/1 -> mech vent mechanics/1
  [Resp_Rhythm] -> Integrator/1, Integrator/2
  Integrator/1 -> Math Function/1
  Math Function/1 -> Transfer Fcn/1
  Transfer Fcn/1 -> Product5/2
  Product5/1 -> Divide/2
  CPAP_activation/1 -> Sum5/2
  Divide/1 -> mech vent neural/1, Sum5/1
  [Mech_Vent_pressure] -> Product5/1
  CPAP Pressure/1(Out1) -> Manual Switch/1
  CPAP_pressure/1 -> Manual Switch/2
  SleepAwake/1 -> Fcn/1
  Fcn/1 -> CPAP_pressure/1
  Manual Switch/1 -> Product/1
  Product/1 -> CPAP_activation/1
  CPAP Control/1(Out1) -> Product/2
  Annoxia or hypercapnia/1(Muscle_Contractility) -> [MuscleContractility]
  [Mech_Vent_activation] -> Divide/1

== system Ventilator_Controller/FVC + Valsalva + Mueller maneuvers ==
  FVC_activation : Constant  Value=FVC_activation
  MEFV Operation : Subsystem  mask{begin_time=t_FVC_start, duration_time=t_FVC_duration, insp_period=t_FVC_insp}
      mask prompts: begin_time "pulse begin"; duration_time "duration"
  Mueller Operation : Subsystem  mask{begin_time=t_Mueller_start, duration_time=t_Mueller_duration, insp_period=t_Mueller_insp}
      mask prompts: begin_time "pulse begin"; duration_time "duration"
  Mueller_activation : Constant  Value=0
  Product{,1..8} (9 alike) : Product  SaturateOnIntegerOverflow=on  InputSameDT=on  OutDataTypeStr=Inherit: Same as first input
  Valsalva Operation : Subsystem  mask{begin_time=t_valsalva_start, duration_time=t_valsalva_duration, insp_period=t_valsalva_insp}
      mask prompts: begin_time "pulse begin"; duration_time "duration"
  Valsalva_activation : Constant  Value=0
  tag scope: FVC_activation=global, FVC_duration=global, FVC_resp_mech=global, FVC_resp_rhythm=global, Mueller_activation=global, Mueller_duration=global, Mueller_resp_mech=global, Mueller_resp_rhythm=global, Valsalva_activation=global, Valsalva_duration=global, Valsalva_resp_mech=global, Valsalva_resp_rhythm=global
  wires:
  Mueller Operation/2(mueller_rhythm) -> Product1/2
  Mueller Operation/3(muller_resp_mech) -> Product2/2
  Mueller Operation/1(duration) -> Product/2
  Product/1 -> [Mueller_duration]
  Product1/1 -> [Mueller_resp_rhythm]
  Product2/1 -> [Mueller_resp_mech]
  Mueller_activation/1 -> Product/1, Product1/1, Product2/1, [Mueller_activation]
  Product3/1 -> [Valsalva_duration]
  Product4/1 -> [Valsalva_resp_rhythm]
  Product5/1 -> [Valsalva_resp_mech]
  Valsalva_activation/1 -> Product3/1, Product4/1, Product5/1, [Valsalva_activation]
  Valsalva Operation/1(duration) -> Product3/2
  Valsalva Operation/2(valsalva_rhythm) -> Product4/2
  Valsalva Operation/3(valsalva_resp_mech) -> Product5/2
  Product6/1 -> [FVC_duration]
  Product7/1 -> [FVC_resp_rhythm]
  Product8/1 -> [FVC_resp_mech]
  FVC_activation/1 -> Product6/1, Product7/1, Product8/1, [FVC_activation]
  MEFV Operation/1(duration) -> Product6/2
  MEFV Operation/2(FVC_rhythm) -> Product7/2
  MEFV Operation/3(FVC_resp_mech) -> Product8/2

== system Ventilator_Controller/Metabolic Control ==
  note: Time Unit: Second
  note: Created by Limei Cheng
  note: Gclamp_in(t)
  Ftas_r : Inport
  SI : Inport  Port=2
  REM : Inport  Port=3
  DIET : Inport  Port=4
  Display & Storage : Subsystem
      mask Display: disp('Display')
  Epinephrine Regulation on Heart and Muscle : Subsystem
  Gain : Subsystem
      mask Display:
      | port_label('output',1,'Glu_Epi')
      | port_label('output',2,'FFA_Epi')
  Glucose Insulin Interventions : Subsystem
  Glucose-Insulin-FFA Minimal Model : Subsystem
  Insulin Clamp : Subsystem
  Sum : Sum  Inputs=|+++  SampleTime=0.6
  Sum1 : Sum  Inputs=|++  SampleTime=0.6
  micromol to mg1 : Gain  Gain=VolG*0.05*10*1*DietBlock  SampleTime=0.6
  micromol to mg2 : Gain  Gain=Keg*(1-Gblock)  SampleTime=0.6
  micromol to mg3 : Gain  Gain=Kef*(1-Gblock)  SampleTime=0.6
  DeltaFtas : Outport
  wires:
  Epinephrine Regulation on Heart and Muscle/1("Epi_Heart Glucose ") -> Gain/1(In1)
  Insulin Clamp/1(Insulin Input) -> Sum1/1
  Epinephrine Regulation on Heart and Muscle/2(Epi_Muscle Glucose) -> Gain/2(In2)
  Epinephrine Regulation on Heart and Muscle/3("Epi_Heart FFA ") -> Gain/3(In3)
  Epinephrine Regulation on Heart and Muscle/4(Epi_Muscle FFA) -> Gain/4(In4)
  Epinephrine Regulation on Heart and Muscle/5(Epi_GI FFA) -> Gain/5(In5)
  Gain/2(F_E) -> micromol to mg3/1  "FFA Input"
  micromol to mg1/1 -> Display & Storage/6(Gin), Sum/2
  Sum/1 -> Glucose-Insulin-FFA Minimal Model/2(u2(t))  "Glucose Input"
  Glucose-Insulin-FFA Minimal Model/1("Plasma Glucose Concn, G(t)") -> Display & Storage/2(G(t)), Glucose Insulin Interventions/1(G(t))
  Glucose-Insulin-FFA Minimal Model/2("Plasma Insulin Concn, I(t)") -> Display & Storage/3(I(t))
  Glucose-Insulin-FFA Minimal Model/3("Plasma FFA Concn, F(t)") -> Display & Storage/4(F(t))
  Epinephrine Regulation on Heart and Muscle/6(Epinephrine Amount Ce(t)) -> Display & Storage/5(E(t))
  Ftas_r/1 -> Epinephrine Regulation on Heart and Muscle/1(Ftas_r)
  SI/1 -> Epinephrine Regulation on Heart and Muscle/2(SI)
  REM/1 -> Epinephrine Regulation on Heart and Muscle/3(REM)
  Glucose-Insulin-FFA Minimal Model/4(DeltaFtas) -> DeltaFtas/1
  DIET/1 -> micromol to mg1/1
  Gain/1(G_E) -> micromol to mg2/1
  micromol to mg3/1 -> Glucose-Insulin-FFA Minimal Model/3(u3(t))
  Sum1/1 -> Display & Storage/1(I(t)_in), Glucose-Insulin-FFA Minimal Model/1(u1(t))
  Glucose Insulin Interventions/1(Glu_in(t)) -> Sum/3
  Glucose Insulin Interventions/3(InsPump_in(t)) -> Sum1/2
  Glucose Insulin Interventions/2(Gclamp_in(t)) -> Display & Storage/7(Gclamp_in)
  Epinephrine Regulation on Heart and Muscle/7(W_alphaSYMP) -> Glucose-Insulin-FFA Minimal Model/4(W_alphaSYMP)
  micromol to mg2/1 -> Sum/1

== system Ventilator_Controller/Progress ==
  t_stop : Inport
  % COMPLETED : Display
      settings: Format=bank
  1/t_end_new : Constant  Value=1/ t_end_new
  100% : Constant  Value=100
  Clock : Clock
  Patient death (ABP<40mmHg) : Subsystem
  Product : Product  SaturateOnIntegerOverflow=on  OutDataTypeStr=Inherit: Same as first input
  Product1 : Product  SaturateOnIntegerOverflow=on  OutDataTypeStr=Inherit: Same as first input
  Relational Operator : RelationalOperator  RndMeth=Nearest  InputSameDT=on
  Rounding Function : Rounding
  SIMULATION DURATION : Display
      settings: Format=bank
  SIMULATION TIME : Display
      settings: Format=bank
  Stop Simulation : Stop
  Stop Simulation1 : Stop
  t_start_new : Constant  Value=t_end_new-t_start_new
  wires:
  t_start_new/1 -> SIMULATION DURATION/1
  Clock/1 -> Relational Operator/1, SIMULATION TIME/1, Product1/1
  Relational Operator/1 -> Stop Simulation/1
  t_stop/1 -> Relational Operator/2
  100%/1 -> Product/2
  1/t_end_new/1 -> Product/1
  Product1/1 -> Rounding Function/1
  Rounding Function/1 -> % COMPLETED/1
  Product/1 -> Product1/2
  Patient death (ABP<40mmHg)/1(Out1) -> Stop Simulation1/1

== system Ventilator_Controller/Respiratory System ==
  Pao : Inport
  Variable Respiratory Rhythm : Inport  Port=2
  RespMus Drive : Inport  Port=3
  Total Ventilatory Drive : Inport  Port=4
  Blood Flow : Inport  Port=5
  Clock : Clock
  Gas Exchange : Subsystem
  Memory : Memory  InheritSampleTime=on
  Modified Upper Airway Conductance : Subsystem
  PE gain : Gain  Gain=30  SaturateOnIntegerOverflow=on  OutDataTypeStr=Inherit: Same as input  ParamDataTypeStr=Inherit: Same as input
  Respiratory_Mechanics : Subsystem  TreatAsAtomicUnit=on
      settings: PropExecContextOutsideSubsystem=on
  Sleep Mechanism : Subsystem
  Sum : Sum  Inputs=-+  SaturateOnIntegerOverflow=on  InputSameDT=on  OutDataTypeStr=Inherit: Same as first input
  Transfer Fcn (with initial outputs) : simulink_extras/Additional Linear/Transfer Fcn (with initial outputs)  N=1  D=[5 1]  Y0=Arousal_CardIC  U0=Arousal_CardIC
  Upper_Airway_Mechanism : Subsystem
  time_span Memory : Memory  InitialCondition=0-time_step
  Tidal Volume (Vt) : Outport
  Sleep/Awake : Outport  Port=2
  PaO2 : Outport  Port=3
  SAO2 : Outport  Port=4
  PbCO2 : Outport  Port=5
  PaCO2 : Outport  Port=6
  CaO2 : Outport  Port=7
  AI - Arousal Index : Outport  Port=8
  SI Sleep Wake State Index : Outport  Port=9
  Pleural Pressure (Ppl) : Outport  Port=10
  REM : Outport  Port=11
  DIET : Outport  Port=12
  tag scope: CONDua=global, Dstate=global, Flow=global, Ppl=global, Vt=global
  wires:
  Respiratory_Mechanics/2(Respiratory Flow) -> Upper_Airway_Mechanism/6(Respiratory Flow Lower Airways), Gas Exchange/3(Air Flow), [Flow]  "Respiratory Flow"
  RespMus Drive/1 -> Respiratory_Mechanics/1("RespMus Drive ")
  PE gain/1 -> Respiratory_Mechanics/3("PE ")
  Total Ventilatory Drive/1 -> Upper_Airway_Mechanism/3(Total Ventilatory Drive)
  Modified Upper Airway Conductance/1(modified upper airway) -> Respiratory_Mechanics/2(Respiratory Conductance)
  Respiratory_Mechanics/1(Vt - Tidal Volume) -> Gas Exchange/1(Vt - Tidal Volume), Upper_Airway_Mechanism/7(Tidal Volume), Tidal Volume (Vt)/1, [Vt]
  Respiratory_Mechanics/3("Ppl ") -> Pleural Pressure (Ppl)/1, [Ppl], Upper_Airway_Mechanism/5(Pleural Pressure)
  Upper_Airway_Mechanism/1(AI - Arousal Index) -> Sleep Mechanism/1(AI - Arousal Index), Transfer Fcn (with initial outputs)/1
  Memory/1 -> Upper_Airway_Mechanism/1(SI Sleep Wake State Index), Gas Exchange/2(SI Sleep Wake State Index)
  Sleep Mechanism/1(SI Sleep Wake State Index) -> Memory/1, [Dstate], SI Sleep Wake State Index/1
  Sleep Mechanism/2(Sleep Awake) -> Upper_Airway_Mechanism/8(Sleep/Awake), Sleep/Awake/1
  Upper_Airway_Mechanism/2("Airway Cond Percentage ") -> [CONDua]
  Gas Exchange/2(PaO2) -> PaO2/1
  Gas Exchange/1(PaCO2) -> PaCO2/1
  Gas Exchange/3(SAO2) -> SAO2/1
  Gas Exchange/4(PbCO2) -> PbCO2/1
  Pao/1 -> Upper_Airway_Mechanism/4(extern pressure), Respiratory_Mechanics/4("Pao ")
  Variable Respiratory Rhythm/1 -> Upper_Airway_Mechanism/2(Variable Respiratory Rhythm)
  Blood Flow/1 -> Gas Exchange/4(Blood Flow)
  [Breathing_Enable] -> Respiratory_Mechanics/Enable
  Sleep Mechanism/3(SWA/S) -> Upper_Airway_Mechanism/9(SWA/S)
  Clock/1 -> time_span Memory/1, Sum/2
  time_span Memory/1 -> Sum/1
  Sum/1 -> Respiratory_Mechanics/5(Step Size), Sleep Mechanism/2(Step_Size)
  Transfer Fcn (with initial outputs)/1 -> AI - Arousal Index/1
  Gas Exchange/5(CaO2) -> CaO2/1
  [Valsalva_resp_mech] -> PE gain/1
  Sleep Mechanism/4(REM) -> REM/1
  Sleep Mechanism/5(Diet1.5h) -> DIET/1

== system Ventilator_Controller/Ventilator control ==
  Ventilator Controller : Subsystem
  tag scope: Mech_Vent_activation=global, Mech_Vent_pressure=global, Mech_Vent_rate=global, NeuroMuscleBlock=global, PIO2=global
  wires:
  [ABP] -> Ventilator Controller/1(ABP)
  [SAO2] -> Ventilator Controller/2(SAO2)
  [Vt] -> Ventilator Controller/3(Vt)
  Ventilator Controller/4(VR) -> [Mech_Vent_rate]
  Ventilator Controller/1(PIO2) -> [PIO2]
  Ventilator Controller/2(NMB) -> [NeuroMuscleBlock]
  Ventilator Controller/5(VP) -> [Mech_Vent_pressure]
  Ventilator Controller/3(VE) -> [Mech_Vent_activation]

== system Ventilator_Controller/Cardiovascular System/Carotid Baroreceptor ==
  ABP : Inport
  "AI - Arousal Index " : Inport  Port=2
  SI Sleep Wake State Index : Inport  Port=3
  Fcn : Fcn  Expr="(exp((u(1) - Pn + (1-u(2)) * u(3) * Pn_sleep ) / (  (1-u(2)) * u(3) *k_cs_sleep + k_cs) ) * fcs_max + fcs_min)/(exp((u(1) - Pn + (1-u(2)) * u(3) * Pn_sleep ) / (  (1-u(2)) * u(3) *k_cs_sleep + k_cs) ) +1) *1"
  Mux : Mux  Inputs=3
  Transfer Fcn : TransferFcn  Numerator=[touz 1]  Denominator=[toup 1]
  fcs : Outport
  wires:
  Fcn/1 -> fcs/1
  Mux/1 -> Fcn/1
  ABP/1 -> Transfer Fcn/1
  "AI - Arousal Index "/1 -> Mux/2
  SI Sleep Wake State Index/1 -> Mux/3
  Transfer Fcn/1 -> Mux/1

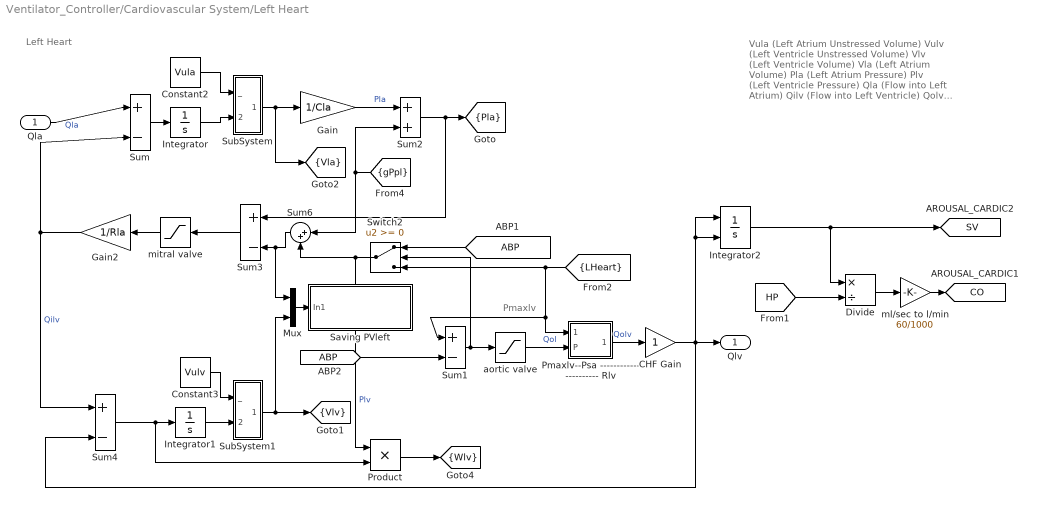
== system Ventilator_Controller/Cardiovascular System/Left Heart ==
  note: Left Heart
  note: Vula (Left Atrium Unstressed Volume)
      | Vulv (Left Ventricle Unstressed Volume)
      | Vlv (Left Ventricle Volume)
      | Vla (Left Atrium Volume)
      | Pla (Left Atrium Pressure)
      | Plv (Left Ventricle Pressure)
      | Qla (Flow into Left Atrium)
      | Qilv (Flow into Left Ventricle)
      | Qolv (Flow out of Left Ventricle)
      | LHeart (Left Ventricle Function)
  note: Pmaxlv
  Qla : Inport
  CHF Gain : Gain
  Constant2 : Constant  Value=Vula
  Constant3 : Constant  Value=Vulv
  Divide : Product  Inputs=*/
  Gain : Gain  Gain=1/Cla  SaturateOnIntegerOverflow=on  OutDataTypeStr=Inherit: Same as input  ParamDataTypeStr=Inherit: Same as input
  Gain2 : Gain  Gain=1/Rla  SaturateOnIntegerOverflow=on  OutDataTypeStr=Inherit: Same as input  ParamDataTypeStr=Inherit: Same as input
  Integrator : Integrator
  Integrator1 : Integrator
  Integrator2 : Integrator  ExternalReset=rising
  Mux : Mux  Inputs=2
  Pmaxlv--Psa ---------------------- Rlv : Subsystem
  Product : Product  RndMeth=Zero
  Saving PVleft : Subsystem
  SubSystem : Subsystem
  SubSystem1 : Subsystem
  Sum : Sum  Inputs=|+-  SaturateOnIntegerOverflow=on  InputSameDT=on  OutDataTypeStr=Inherit: Same as first input
  Sum1 : Sum  Inputs=+-  SaturateOnIntegerOverflow=on  InputSameDT=on  OutDataTypeStr=Inherit: Same as first input
  Sum2 : Sum  SaturateOnIntegerOverflow=on  InputSameDT=on  OutDataTypeStr=Inherit: Same as first input
  Sum3 : Sum  Inputs=+-  SaturateOnIntegerOverflow=on  InputSameDT=on  OutDataTypeStr=Inherit: Same as first input
  Sum4 : Sum  Inputs=+-  SaturateOnIntegerOverflow=on  InputSameDT=on  OutDataTypeStr=Inherit: Same as first input
  Sum6 : Sum  Inputs=|++
  Switch2 : Switch  SaturateOnIntegerOverflow=on  InputSameDT=on
  aortic valve : Saturate  UpperLimit=inf  LowerLimit=0
  mitral valve : Saturate  UpperLimit=inf  LowerLimit=0
  ml/sec to l/min : Gain  Gain=60/1000
  Qlv : Outport
  tag scope: CO=global, Pla=scoped, SV=global, Vla=scoped, Vlv=scoped, Wlv=scoped
  wires:
  Qla/1 -> Sum/1  "Qla"
  Sum/1 -> Integrator/1
  [ABP] -> Sum1/2
  Sum4/1 -> Integrator1/1, Product/2
  Gain2/1 -> Sum/2, Sum4/1  "Qilv"
  Pmaxlv--Psa ---------------------- Rlv/1(Flow) -> CHF Gain/1  "Qolv"
  Constant2/1 -> SubSystem/1(_)
  Constant3/1 -> SubSystem1/1(_)
  SubSystem/1(Out) -> Gain/1, [Vla]
  Sum1/1 -> aortic valve/1, Switch2/2
  [ABP] -> Switch2/1
  mitral valve/1 -> Gain2/1
  [LHeart] -> Switch2/3, Pmaxlv--Psa ---------------------- Rlv/1(Pmax), Sum1/1
  aortic valve/1 -> Pmaxlv--Psa ---------------------- Rlv/2(P)  "Qol"
  SubSystem1/1(Out) -> Mux/2, [Vlv]
  Integrator1/1 -> SubSystem1/2(+)
  Sum3/1 -> mitral valve/1
  Integrator/1 -> SubSystem/2(+)
  Gain/1 -> Sum2/1  "Pla"
  Sum2/1 -> [Pla], Sum3/1
  Switch2/1 -> Sum6/2, Product/1  "Plv"
  Sum6/1 -> Sum3/2, Mux/1
  [gPpl] -> Sum2/2, Sum6/1
  Product/1 -> [Wlv]
  CHF Gain/1 -> Qlv/1, Integrator2/2, Integrator2/1, Sum4/2
  Divide/1 -> ml/sec to l/min/1
  [HP] -> Divide/2
  Integrator2/1 -> Divide/1, [SV]
  ml/sec to l/min/1 -> [CO]
  Mux/1 -> Saving PVleft/1(In1)

== system Ventilator_Controller/Cardiovascular System/Local Flow Regulation ==
  AI (arousal  Index) : Inport
  "SI (Sleep Index) " : Inport  Port=2
  PaCO2 : Inport  Port=3
  CaO2 : Inport  Port=4
  Qmp : Inport  Port=5
  Qbp : Inport  Port=6
  Qhp : Inport  Port=7
  Cerebral Circulation Regulation : Subsystem
  Coronary Circulation Regulation2 : Subsystem
  Fcn1 : Fcn  Expr=1-u
  Gas_sleep : Gain  Gain=Gas_sleep  SaturateOnIntegerOverflow=on  OutDataTypeStr=Inherit: Same as input  ParamDataTypeStr=Inherit: Same as input
  Muscular Circulation Regulation1 : Subsystem
  Product2 : Product  SaturateOnIntegerOverflow=on  InputSameDT=on  OutDataTypeStr=Inherit: Same as first input
  Sum3 : Sum  Inputs=-+  SaturateOnIntegerOverflow=on  InputSameDT=on  OutDataTypeStr=Inherit: Same as first input
  constant : Constant
  tag scope: Gbp=scoped, Rhp=scoped, Rmp=scoped
  wires:
  CaO2/1 -> Cerebral Circulation Regulation/1(CaO2), Muscular Circulation Regulation1/1(CaO2), Coronary Circulation Regulation2/1(CaO2)
  PaCO2/1 -> Cerebral Circulation Regulation/2(PaCO2), Muscular Circulation Regulation1/2(PaCO2), Coronary Circulation Regulation2/2(PaCO2)
  Cerebral Circulation Regulation/1(Gbp) -> [Gbp]
  Muscular Circulation Regulation1/1(Rmp) -> [Rmp]
  Coronary Circulation Regulation2/1(Rhp) -> [Rhp]
  Qbp/1 -> Cerebral Circulation Regulation/3(Qbp)
  Qmp/1 -> Muscular Circulation Regulation1/3(Qmp)
  Qhp/1 -> Coronary Circulation Regulation2/3(Qhp)
  AI (arousal  Index)/1 -> Fcn1/1
  "SI (Sleep Index) "/1 -> Product2/2
  Fcn1/1 -> Product2/1
  Product2/1 -> Gas_sleep/1
  constant/1 -> Sum3/2
  Gas_sleep/1 -> Sum3/1
  Sum3/1 -> Coronary Circulation Regulation2/4(Gsleep), Muscular Circulation Regulation1/4(Gsleep), Cerebral Circulation Regulation/4(Gsleep)  "Gas(SI)"

== system Ventilator_Controller/Cardiovascular System/Pulmonary ==
  note: Ppa (Pulmonary Arteries Pressure)
      | Ppp (Pulmonary Peripheral Pressure)
      | Ppv (Pulmonary Veins Pressure)
      | Pla (Left Atrium Pressure)
      | Qor (Flow from Right Heart)
      | Qpa (Flow to Pulmonary Aorta)
      | Qla (Flow to Left Atrium)
      | Vupa (Pulmonary Arteries Unstressed Volume)
      | Vupp (Pulmonary Peripheral Unstressed Volume)
      | Vupv (Pulmonary Veins Unstressed Volume)
  note: Pulmonary Circulation
  Qrv : Inport
  Constant : Constant  Value=Vupa
  Constant1 : Constant  Value=Vupp
  Constant3 : Constant  Value=Vupv
  Gain : Gain  Gain=1/Cpa  SaturateOnIntegerOverflow=on  OutDataTypeStr=Inherit: Same as input  ParamDataTypeStr=Inherit: Same as input
  Gain1 : Gain  Gain=1/Lpa  SaturateOnIntegerOverflow=on  OutDataTypeStr=Inherit: Same as input  ParamDataTypeStr=Inherit: Same as input
  Gain2 : Gain  Gain=Rpa  SaturateOnIntegerOverflow=on  OutDataTypeStr=Inherit: Same as input  ParamDataTypeStr=Inherit: Same as input
  Gain4 : Gain  Gain=1/Rpp  SaturateOnIntegerOverflow=on  OutDataTypeStr=Inherit: Same as input  ParamDataTypeStr=Inherit: Same as input
  Gain5 : Gain  Gain=1/Cpp  SaturateOnIntegerOverflow=on  OutDataTypeStr=Inherit: Same as input  ParamDataTypeStr=Inherit: Same as input
  Gain6 : Gain  Gain=1/Cpv  SaturateOnIntegerOverflow=on  OutDataTypeStr=Inherit: Same as input  ParamDataTypeStr=Inherit: Same as input
  Gain7 : Gain  Gain=1/Rpv  SaturateOnIntegerOverflow=on  OutDataTypeStr=Inherit: Same as input  ParamDataTypeStr=Inherit: Same as input
  Integrator : Integrator  InitialCondition=100
  Integrator1 : Integrator
  Integrator2 : Integrator  InitialCondition=100
  Integrator3 : Integrator
  SubSystem : Subsystem
  SubSystem1 : Subsystem
  SubSystem2 : Subsystem
  Sum{,2,4..5} (4 alike) : Sum  Inputs=+-  SaturateOnIntegerOverflow=on  InputSameDT=on  OutDataTypeStr=Inherit: Same as first input
  Sum1 : Sum  Inputs=-+-  SaturateOnIntegerOverflow=on  InputSameDT=on  OutDataTypeStr=Inherit: Same as first input
  Sum3 : Sum  Inputs=++-  SaturateOnIntegerOverflow=on  InputSameDT=on  OutDataTypeStr=Inherit: Same as first input
  Sum6 : Sum  Inputs=|++
  Sum7 : Sum
  ml/liter : Gain  Gain=1/1000  SaturateOnIntegerOverflow=on  OutDataTypeStr=Inherit: Same as input  ParamDataTypeStr=Inherit: Same as input
  Qpp : Outport
  Qla : Outport  Port=2
  tag scope: Ppa=scoped, Vpa=scoped, Vpp=scoped, Vpv=scoped
  wires:
  Qrv/1 -> Sum/1  "Qrv"
  Sum/1 -> Integrator/1
  Integrator1/1 -> Gain1/1
  Sum1/1 -> Integrator1/1
  Gain2/1 -> Sum1/3
  Gain1/1 -> Sum/2, Gain2/1, Sum2/1  "Qpa"
  Sum2/1 -> Integrator2/1
  Gain5/1 -> Sum1/1, Sum3/1  "Ppp"
  Sum3/1 -> Gain4/1
  Gain4/1 -> Sum2/2, Sum4/1, ml/liter/1
  Sum5/1 -> Gain7/1
  [Pla] -> Sum5/2  "Pla"
  Sum4/1 -> Integrator3/1  "Fla"
  SubSystem/1(Out) -> Gain/1, [Vpa]
  SubSystem1/1(Out) -> Gain5/1, [Vpp]
  SubSystem2/1(Out) -> Gain6/1, [Vpv]
  Integrator/1 -> SubSystem/2(+)
  Constant/1 -> SubSystem/1(_)
  Constant1/1 -> SubSystem1/1(_)
  Integrator2/1 -> SubSystem1/2(+)
  Integrator3/1 -> SubSystem2/2(+)
  Gain7/1 -> Qla/1, Sum4/2  "Qpv"
  Constant3/1 -> SubSystem2/1(_)
  Gain/1 -> Sum6/1  "Ppa"
  Sum6/1 -> Sum1/2, [Ppa]
  Gain6/1 -> Sum7/2  "Ppv"
  Sum7/1 -> Sum5/1, Sum3/3
  [gPpl] -> Sum7/1, Sum3/2
  ml/liter/1 -> Qpp/1
  [gPpl] -> Sum6/2
